simulink model "sampleModel58"  (R2021b)
settings: Solver=VariableStepAuto  StartTime=0.0  StopTime=10.0  RelTol=1e-3
libraries: simulink x6
settings Model: Creator=user  LastModifiedBy=user

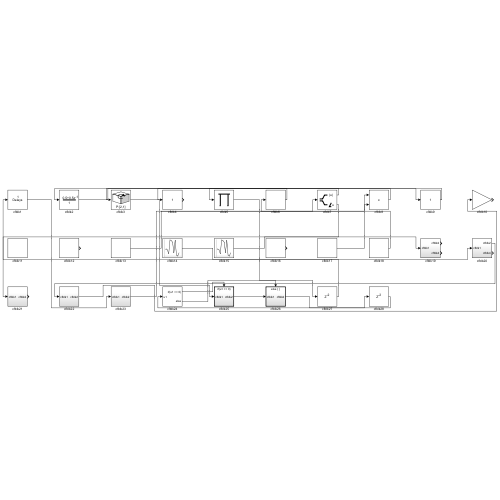
[thumbnail: Simulink's stored preview of the top-level diagram]
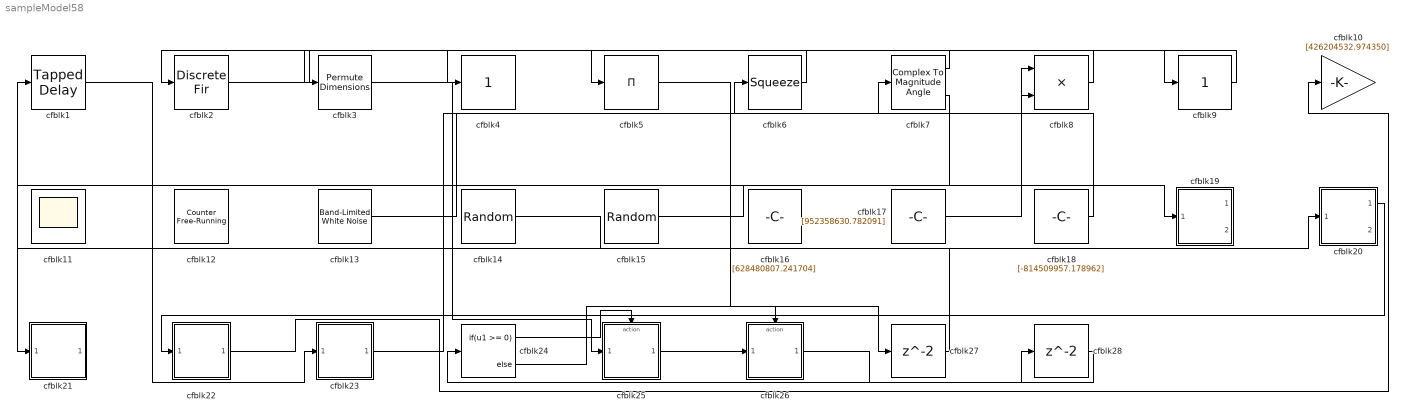
== system sampleModel58 ==
  cfblk1 : simulink/Discrete/Tapped Delay  vinit=0.0  samptime=-1  NumDelays=1  DelayOrder=Oldest  includeCurrent=off
  cfblk10 : Gain  Gain=[426204532.974350]
  cfblk11 : Scope
      settings: Floating=on
  cfblk12 : simulink/Sources/Counter Free-Running  NumBits=[44.000000]  tsamp=-1
  cfblk13 : simulink/Sources/Band-Limited White Noise  Cov=[8884358361.139034]  Ts=0.1  seed=[5389175955.000000]
  cfblk14 : RandomNumber  Mean=[-61685.528728]  Variance=[77249.203375]  Seed=[618355507.000000]  SampleTime=0.1
  cfblk15 : RandomNumber  Mean=[87699.194747]  Variance=[49189.128423]  Seed=[354297291.000000]  SampleTime=0.1
  cfblk16 : Constant  Value=[628480807.241704]  SampleTime=1
  cfblk17 : Constant  Value=[952358630.782091]  SampleTime=1
  cfblk18 : Constant  Value=[-814509957.178962]  SampleTime=1
  cfblk19 : Subsystem
  cfblk2 : DiscreteFir  SampleTime=1
  cfblk20 : Subsystem
  cfblk21 : Subsystem
  cfblk22 : Subsystem
  cfblk23 : Subsystem
  cfblk24 : If  IfExpression=u1 >= 0  SampleTime=1
  cfblk25 : Subsystem  TreatAsAtomicUnit=on
  cfblk26 : Subsystem  TreatAsAtomicUnit=on
  cfblk27 : Delay  SampleTime=1
  cfblk28 : Delay  SampleTime=1
  cfblk3 : PermuteDimensions
  cfblk4 : simulink/Math Operations/Slider Gain  gain=1  low=0  high=2
  cfblk5 : Product  Inputs=*
  cfblk6 : Squeeze
  cfblk7 : ComplexToMagnitudeAngle
  cfblk8 : Product  Inputs=**
  cfblk9 : simulink/Math Operations/Slider Gain  gain=1  low=0  high=2
  wires:
  cfblk20/1(cfblk2) -> cfblk22/1(cfblk1)
  cfblk15/1 -> cfblk19/1(cfblk1)
  cfblk1/1 -> cfblk23/1(cfblk1)
  cfblk22/1(cfblk2) -> cfblk10/1
  cfblk18/1 -> cfblk6/1
  cfblk23/1(cfblk2) -> cfblk7/1
  cfblk13/1 -> cfblk8/1
  cfblk7/1 -> cfblk2/1
  cfblk3/1 -> cfblk25/1(cfblk1)
  cfblk17/1 -> cfblk8/2
  cfblk2/1 -> cfblk9/1
  cfblk7/2 -> cfblk21/1(cfblk1)
  cfblk6/1 -> cfblk4/1
  cfblk14/1 -> cfblk20/1(cfblk1)
  cfblk8/1 -> cfblk3/1
  cfblk9/1 -> cfblk5/1
  cfblk25/1(cfblk2) -> cfblk26/1(cfblk1)
  cfblk24/1 -> cfblk25/Action
  cfblk24/2 -> cfblk26/Action
  cfblk5/1 -> cfblk27/1
  cfblk27/1 -> cfblk1/1
  cfblk26/1(cfblk2) -> cfblk28/1
  cfblk28/1 -> cfblk24/1

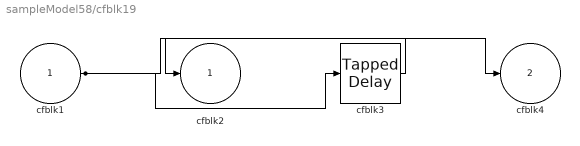
== system sampleModel58/cfblk19 ==
  cfblk1 : Inport
  cfblk3 : simulink/Discrete/Tapped Delay  vinit=0.0  samptime=-1  NumDelays=1  DelayOrder=Oldest  includeCurrent=off
  cfblk2 : Outport
  cfblk4 : Outport  Port=2
  wires:
  cfblk3/1 -> cfblk2/1
  cfblk1/1 -> cfblk3/1, cfblk4/1

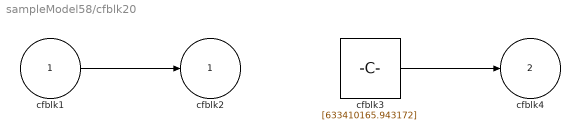
== system sampleModel58/cfblk20 ==
  cfblk1 : Inport
  cfblk3 : Constant  Value=[633410165.943172]  SampleTime=1
  cfblk2 : Outport
  cfblk4 : Outport  Port=2
  wires:
  cfblk1/1 -> cfblk2/1
  cfblk3/1 -> cfblk4/1

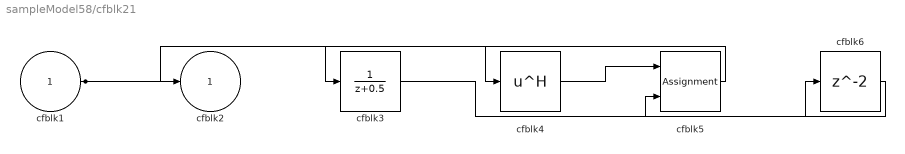
== system sampleModel58/cfblk21 ==
  cfblk1 : Inport
  cfblk3 : DiscreteTransferFcn  SampleTime=1
  cfblk4 : Math  Operator=hermitian  SaturateOnIntegerOverflow=on
  cfblk5 : Assignment  DiagnosticForDimensions=Warning  IndexOptions=Index vector (dialog)  Indices=1  OutputSizes=1
  cfblk6 : Delay  SampleTime=1
  cfblk2 : Outport
  wires:
  cfblk5/1 -> cfblk3/1
  cfblk4/1 -> cfblk5/1
  cfblk1/1 -> cfblk2/1, cfblk4/1
  cfblk3/1 -> cfblk6/1
  cfblk6/1 -> cfblk5/2

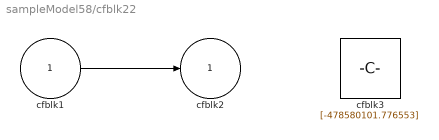
== system sampleModel58/cfblk22 ==
  cfblk1 : Inport
  cfblk3 : Constant  Value=[-478580101.776553]  SampleTime=1
  cfblk2 : Outport
  wires:
  cfblk1/1 -> cfblk2/1

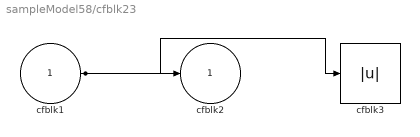
== system sampleModel58/cfblk23 ==
  cfblk1 : Inport
  cfblk3 : Abs
  cfblk2 : Outport
  wires:
  cfblk1/1 -> cfblk2/1, cfblk3/1

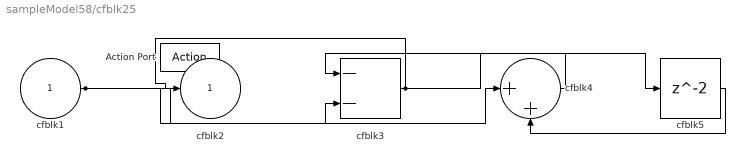
== system sampleModel58/cfblk25 ==
  cfblk1 : Inport
  Action Port : ActionPort  ActionPortLabel=if(u1 >= 0)
  cfblk3 : Sum  Inputs=--
  cfblk4 : Sum  Inputs=|++
  cfblk5 : Delay
  cfblk2 : Outport
  wires:
  cfblk1/1 -> cfblk4/1, cfblk3/2
  cfblk3/1 -> cfblk2/1, cfblk5/1
  cfblk4/1 -> cfblk3/1
  cfblk5/1 -> cfblk4/2

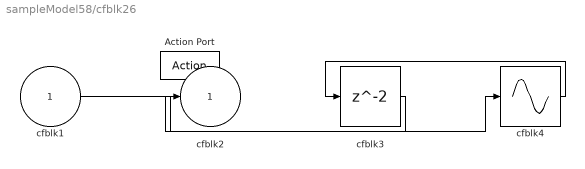
== system sampleModel58/cfblk26 ==
  cfblk1 : Inport
  Action Port : ActionPort  ActionPortLabel=else
  cfblk3 : Delay
  cfblk4 : Sin  TimeSource=Use external signal  SampleTime=0
  cfblk2 : Outport
  wires:
  cfblk1/1 -> cfblk4/1
  cfblk4/1 -> cfblk3/1
  cfblk3/1 -> cfblk2/1
